simulink model "Integral_cntrl_ex2"  (R2023a)
settings: Solver=VariableStepAuto  StartTime=0.0  StopTime=10  RelTol=1e-3
values from neighbouring files (symbols this model uses):
  Ad = SYSd.A    [dual_param.m]    (also in dual_param_ex3.m)
  Bd = SYSd.B    [dual_param.m]    (also in dual_param_ex3.m)
  Cd = SYSd.C    [dual_param.m]    (also in dual_param_ex3.m)
  Nu = N1(n+1:n+m,1:r)    [dual_param.m]    (also in dual_param_ex3.m)
  Nx = N1(1:n,1:r)    [dual_param.m]    (also in dual_param_ex3.m)
  Ts = 10E-3    (= 0.01)    [dual_param.m]    (also in dual_param_ex3.m)
undefined symbols (not defined in the file or in its folder): K
settings Model: Creator=Admin  LastModifiedBy=Admin
settings ModelReferenceCC: EnableRefExpFcnMdlSchedulingChecks=on

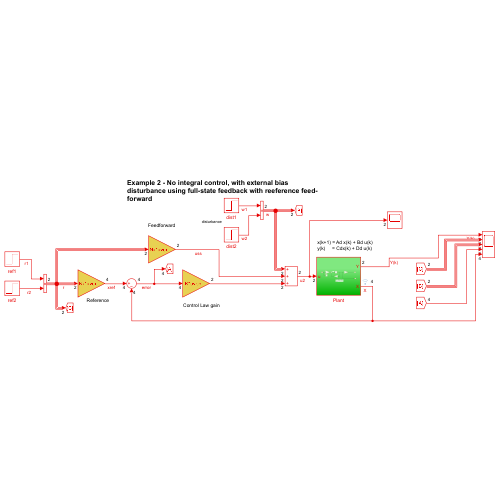
[thumbnail: Simulink's stored preview of the top-level diagram]
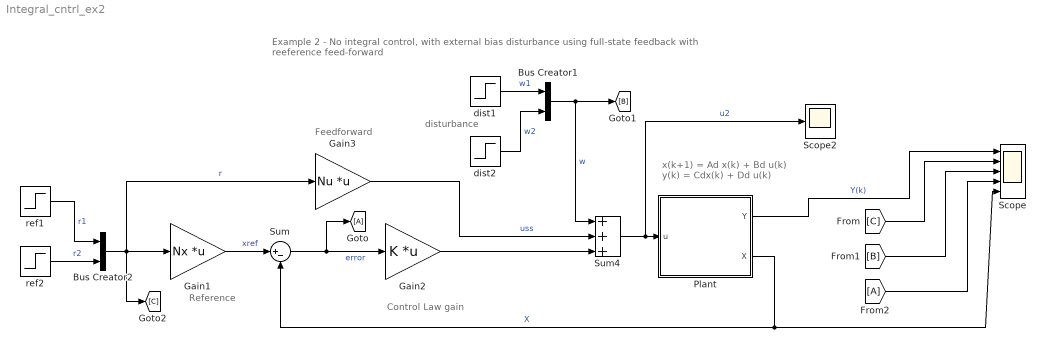
== system Integral_cntrl_ex2 ==
  note: Reference
  note: Feedforward
  note: Example 2 - No integral control, with external bias disturbance using full-state feedback with reeference feed-forward
  note: disturbance
  note: Control Law gain
  note: x(k+1) = Ad x(k) + Bd u(k)
      | y(k)     = Cdx(k) + Dd u(k)
  Bus Creator1 : BusCreator  Inputs=2
  Bus Creator2 : BusCreator  Inputs=2
  From2 : From
  Gain1 : Gain  Gain=Nx  Multiplication=Matrix(K*u) (u vector)
  Gain2 : Gain  Gain=K  Multiplication=Matrix(K*u) (u vector)
  Gain3 : Gain  Gain=Nu  Multiplication=Matrix(K*u) (u vector)
  Goto : Goto
  Plant : Subsystem
  Scope : Scope  NumInputPorts=5
  Scope2 : Scope
  Sum : Sum  Inputs=|+-
  Sum4 : Sum  Inputs=+++
  dist1 : Step  Time=6  SampleTime=Ts
  dist2 : Step  Time=10  After=0  SampleTime=Ts
  ref1 : Step  Time=0  After=2  SampleTime=Ts
  ref2 : Step  Time=3.0  After=1.5  SampleTime=Ts
  wires:
  Sum/1 -> Gain2/1, Goto/1  "error"
  Plant/1(Y) -> Scope/1  "Y(k)"
  [C] -> Scope/2
  [B] -> Scope/3
  dist1/1 -> Bus Creator1/1  "w1"
  ref1/1 -> Bus Creator2/1  "r1"
  ref2/1 -> Bus Creator2/2  "r2"
  Bus Creator2/1 -> Gain3/1, Gain1/1, [C]  "r"
  dist2/1 -> Bus Creator1/2  "w2"
  Sum4/1 -> Scope2/1, Plant/1(u)  "u2"
  Bus Creator1/1 -> [B], Sum4/1  "w"
  From2/1 -> Scope/4
  Gain1/1 -> Sum/1  "xref"
  Plant/2(X) -> Scope/5, Sum/2  "X"
  Gain2/1 -> Sum4/3
  Gain3/1 -> Sum4/2  "uss"

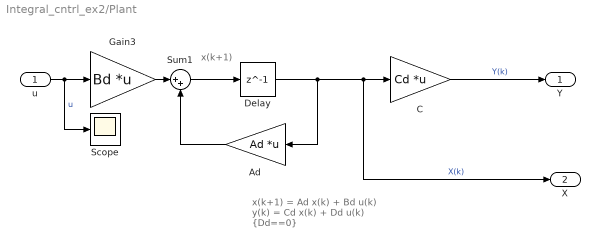
== system Integral_cntrl_ex2/Plant ==
  note: x(k+1) = Ad x(k) + Bd u(k)
      | y(k) = Cd x(k) + Dd u(k) {Dd==0}
  note: x(k+1)
  u : Inport
  Ad : Gain  Gain=Ad  Multiplication=Matrix(K*u) (u vector)
  C : Gain  Gain=Cd  Multiplication=Matrix(K*u) (u vector)
  Delay : Delay  DelayLength=1
  Gain3 : Gain  Gain=Bd  Multiplication=Matrix(K*u) (u vector)
  Scope : Scope
  Sum1 : Sum  Inputs=|++
  Y : Outport
  X : Outport  Port=2
  wires:
  u/1 -> Scope/1, Gain3/1  "u"
  Sum1/1 -> Delay/1
  Delay/1 -> Ad/1, X/1, C/1  "X(k)"
  Gain3/1 -> Sum1/1
  Ad/1 -> Sum1/2
  C/1 -> Y/1  "Y(k)"
